simulink model "model_PMM_ph_gaslift"  (R2023a)
settings: Solver=ode15s  StartTime=0  StopTime=par.simulation_time  FixedStep=par.sample_time  RelTol=1e-3
values from neighbouring files (symbols this model uses):
  par = function_parameters_MPC_PMM_ph_gaslift    [main_MPC_PMM_ph_gaslift.m]
settings Model: Creator=aslik  LastModifiedBy=aslik
settings SolverCC: ZeroCrossAlgorithm=Adaptive
settings DataIOCC: SignalLogging=off  ReturnWorkspaceOutputs=off  DatasetSignalFormat=timetable
settings OptimizationCC: BlockReduction=off  OptimizeBlockIOStorage=off  BufferReuse=off
settings DebuggingCC: AlgebraicLoopMsg=none
settings ModelReferenceCC: EnableRefExpFcnMdlSchedulingChecks=on
settings RTWCC: DLArmComputeVersion=19.05

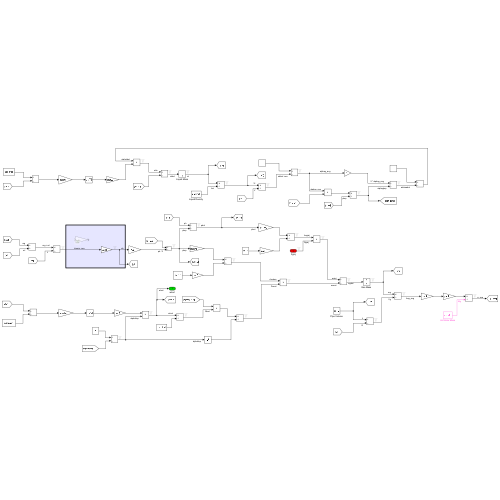
[thumbnail: Simulink's stored preview of the top-level diagram]
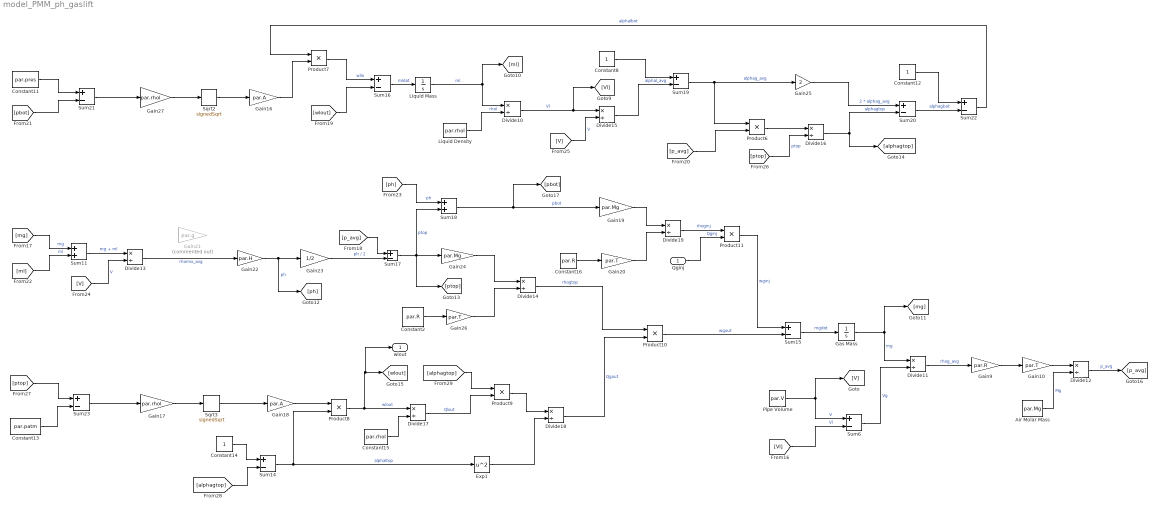
== system model_PMM_ph_gaslift ==
  Qginj : Inport
  Air Molar Mass : Constant  Value=par.Mg  OutDataTypeStr=double
  Constant11 : Constant  Value=par.pres  OutDataTypeStr=double
  Constant12 : Constant  OutDataTypeStr=double
  Constant13 : Constant  Value=par.patm  OutDataTypeStr=double
  Constant14 : Constant  OutDataTypeStr=double
  Constant15 : Constant  Value=par.rhol  OutDataTypeStr=double
  Constant16 : Constant  Value=par.R  OutDataTypeStr=double
  Constant2 : Constant  Value=par.R  OutDataTypeStr=double
  Constant8 : Constant  OutDataTypeStr=double
  Divide{10..19} (10 alike) : Product  Inputs=*/
  Exp1 : Math  Operator=square
  Gain10 : Gain  Gain=par.T
  Gain16 : Gain  Gain=par.A
  Gain17 : Gain  Gain=par.rhol
  Gain18 : Gain  Gain=par.A
  Gain19 : Gain  Gain=par.Mg
  Gain20 : Gain  Gain=par.T
  Gain21 : Gain  Commented=on  Gain=par.g
  Gain22 : Gain  Gain=par.H
  Gain23 : Gain  Gain=1/2
  Gain24 : Gain  Gain=par.Mg
  Gain25 : Gain  Gain=2
  Gain26 : Gain  Gain=par.T
  Gain27 : Gain  Gain=par.rhol
  Gain9 : Gain  Gain=par.R
  "Gas Mass " : Integrator  InitialCondition=par.mg0  LowerSaturationLimit=0  ContinuousStateAttributes='mg'
  Liquid Density : Constant  Value=par.rhol  OutDataTypeStr=double
  Liquid Mass : Integrator  InitialCondition=par.ml0  LowerSaturationLimit=0  ContinuousStateAttributes='ml'
  Pipe Volume : Constant  Value=par.V  OutDataTypeStr=double
  Product{6..11} (6 alike) : Product
  Sqrt2 : Sqrt  Operator=signedSqrt
  Sqrt3 : Sqrt  Operator=signedSqrt
  Sum11 : Sum
  Sum{6,14..17,19..23} (10 alike) : Sum  Inputs=+-
  Sum18 : Sum
  wlout : Outport
  wires:
  Sum19/1 -> Product6/1, Gain25/1  "alphag_avg"
  Constant2/1 -> Gain26/1
  Gain18/1 -> Product8/1
  Product10/1 -> Sum15/2  "wgout"
  Constant13/1 -> Sum23/2
  Sum6/1 -> Divide11/2  "Vg"
  Liquid Density/1 -> Divide10/2  "rhol"
  Sum11/1 -> Divide13/1  "mg + ml"
  Liquid Mass/1 -> [ml], Divide10/1  "ml"
  Gain17/1 -> Sqrt3/1
  [mg] -> Sum11/1  "mg"
  Gain22/1 -> [ph], Gain23/1  "ph"
  [pbot] -> Sum21/2
  Sum20/1 -> Sum22/2  "alphagbot"
  Sum18/1 -> [pbot], Gain19/1  "pbot"
  Air Molar Mass/1 -> Divide12/2  "Mg"
  Product9/1 -> Divide18/1
  [V] -> Divide13/2  "V"
  [wlout] -> Sum16/2
  [ml] -> Sum11/2  "ml"
  [p_avg] -> Sum17/1
  [Vl] -> Sum6/2  "Vl"
  Sum21/1 -> Gain27/1
  Gain10/1 -> Divide12/1
  Gain20/1 -> Divide19/2
  Pipe Volume/1 -> [V], Sum6/1  "V"
  [ptop] -> Divide16/2  "ptop"
  Exp1/1 -> Divide18/2
  Divide18/1 -> Product10/2  "Qgout"
  Constant12/1 -> Sum22/1
  Gain23/1 -> Sum17/2  "ph / 2"
  Gain9/1 -> Gain10/1
  Qginj/1 -> Product11/2  "Qginj"
  Sum15/1 -> "Gas Mass "/1  "mgdot"
  [alphagtop] -> Product9/1
  Gain19/1 -> Divide19/1
  Constant15/1 -> Divide17/2
  Sum23/1 -> Gain17/1
  Constant14/1 -> Sum14/1
  Divide12/1 -> [p_avg]  "p_avg"
  Gain16/1 -> Product7/2
  Gain27/1 -> Sqrt2/1
  Product6/1 -> Divide16/1
  Gain24/1 -> Divide14/1
  Divide10/1 -> Divide15/1, [Vl]  "Vl"
  [ptop] -> Sum23/1
  Divide17/1 -> Product9/2  "Qlout"
  [ph] -> Sum18/1  "ph"
  Sum14/1 -> Product8/2, Exp1/1  "alphaltop"
  Divide16/1 -> [alphagtop], Sum20/2  "alphagtop"
  Constant16/1 -> Gain20/1
  Gain26/1 -> Divide14/2
  "Gas Mass "/1 -> [mg], Divide11/1  "mg"
  Sum22/1 -> Product7/1  "alphalbot"
  [alphagtop] -> Sum14/2
  Product8/1 -> wlout/1, [wlout], Divide17/1  "wlout"
  Divide11/1 -> Gain9/1  "rhog_avg"
  [p_avg] -> Product6/2
  Product11/1 -> Sum15/1  "wginj"
  Constant8/1 -> Sum19/1
  Sum16/1 -> Liquid Mass/1  "mldot"
  Constant11/1 -> Sum21/1
  [V] -> Divide15/2  "V"
  Divide13/1 -> Gain22/1  "rhomix_avg"
  Product7/1 -> Sum16/1  "wlin"
  Divide15/1 -> Sum19/2  "alphal_avg"
  Sum17/1 -> Gain24/1, Sum18/2, [ptop]  "ptop"
  Gain25/1 -> Sum20/1  "2 * alphag_avg"
  Divide14/1 -> Product10/1  "rhogtop"
  Divide19/1 -> Product11/1  "rhoginj"
  Sqrt3/1 -> Gain18/1
  Sqrt2/1 -> Gain16/1
